simulink model "taller3"  (R2026a)
settings: Solver=VariableStepAuto  StopTime=20.0
libraries: simulink x2, slpidlib x1
settings Model: Creator=User  LastModifiedBy=User

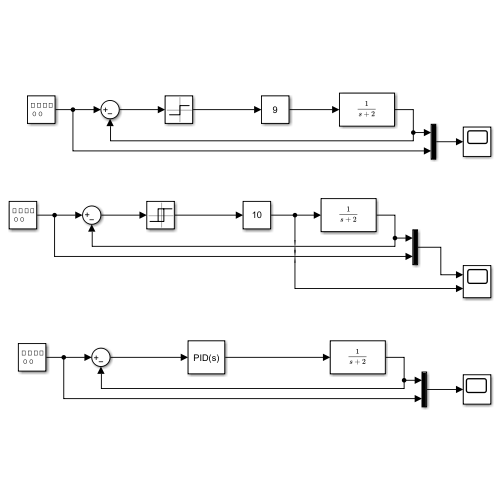
[thumbnail: Simulink's stored preview of the top-level diagram]
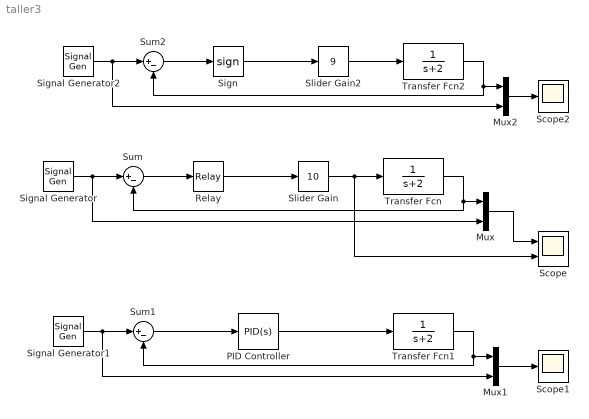
== system taller3 ==
  Mux : Mux  Inputs=2
  Mux1 : Mux  Inputs=2
  Mux2 : Mux  Inputs=2
  PID Controller : slpidlib/PID Controller  Controller=PID  Form=Parallel  TimeDomain=Continuous-time  UseExternalTs=off  SampleTime=-1  IntegratorMethod=Forward Euler  FilterMethod=Forward Euler  ControllerParametersSource=internal  P=50  I=0.5  UseKiTs=off  D=1  UseExternalDerivativeSource=off  N=100  UseFilter=on  TunerSelectOption=Transfer Function Based (PID Tuner App)  ZeroCross=off  InitialConditionSource=internal  InitialConditionForIntegrator=0  InitialConditionForFilter=0  DifferentiatorICPrevScaledInput=0  ExternalReset=none  TrackingMode=off  Kt=1  LimitOutput=off  SatLimitsSource=internal  UpperSaturationLimit=inf  LowerSaturationLimit=-inf  LinearizeAsGain=on  AntiWindupMode=none  Kb=1  LimitIntegrator=off  UpperIntegratorSaturationLimit=inf  LowerIntegratorSaturationLimit=-inf  POutMin=[]  POutMax=[]  IOutMin=[]  IOutMax=[]  DOutMin=[]  DOutMax=[]  NOutMin=[]  NOutMax=[]  SumOutMin=[]  SumOutMax=[]  SaturationOutMin=[]  SaturationOutMax=[]  PParamMin=[]  PParamMax=[]  IParamMin=[]  IParamMax=[]  DParamMin=[]  DParamMax=[]  NParamMin=[]  NParamMax=[]  KbParamMin=[]  KbParamMax=[]  KtParamMin=[]  KtParamMax=[]  KbOutMin=[]  KbOutMax=[]  KtOutMin=[]  KtOutMax=[]  IntegratorOutMin=[]  IntegratorOutMax=[]  FilterOutMin=[]  FilterOutMax=[]  SumI1OutMin=[]  SumI1OutMax=[]  SumI2OutMin=[]  SumI2OutMax=[]  SumI3OutMin=[]  SumI3OutMax=[]  SumI4OutMin=[]  SumI4OutMax=[]  SumDOutMin=[]  SumDOutMax=[]  DifferentiatorOutMin=[]  DifferentiatorOutMax=[]  FilterDiffOutCoefMin=[]  FilterDiffOutCoefMax=[]  ReciprocalOutMin=[]  ReciprocalOutMax=[]  SumDenOutMin=[]  SumDenOutMax=[]  SumNumOutMin=[]  SumNumOutMax=[]  DivideOutMin=[]  DivideOutMax=[]  UdiffTsProdOutMin=[]  UdiffTsProdOutMax=[]  NTsProdOutMin=[]  NTsProdOutMax=[]  UintegralTsProdOutMin=[]  UintegralTsProdOutMax=[]  UngainTsProdOutMin=[]  UngainTsProdOutMax=[]  ClampingZeroOutDataTypeStr=Inherit: Inherit via back propagation  ClampingZeroOutMin=[]  ClampingZeroOutMax=[]  FilterDenConstantOutDataTypeStr=Inherit: Inherit via back propagation  FilterDenConstantOutMin=[]  FilterDenConstantOutMax=[]  PCopyOutDataTypeStr=Inherit: Inherit via back propagation  PCopyOutMin=[]  PCopyOutMax=[]  NCopyOutDataTypeStr=Inherit: Inherit via back propagation  NCopyOutMin=[]  NCopyOutMax=[]  IntegratorContinuousStateAttributes=''  IntegratorStateMustResolveToSignalObject=off  IntegratorRTWStateStorageClass=Auto  FilterContinuousStateAttributes=''  FilterStateMustResolveToSignalObject=off  FilterRTWStateStorageClass=Auto  ParallelPVariant=InternalParameters  IdealPVariant=Disabled  IVariant=InternalParameters  DVariant=InternalParameters  IntegratorVariant=Continuous  SatVariant=Disabled  AWVariant=Passthrough  PCopyVariant=Disabled  TRVariant=Disabled  FdbkBlocksVariant=Forward  IdealPFdbkVariant=Disabled  SatFdbkVariant=Disabled  DerivativeFilterVariant=ContFilter  NVariant=InternalParameters  NCopyVariant=Disabled  FilterICVariant=InternalICsFilter  IntegratorICVariant=InternalICs  ExternalResetVariant=Disabled  TRSumVariant=Passthrough  SumFdbkVariant=Disabled  SumVariant=Sum_PID  TsampFilterVariant=InternalTs  TsampNgainVariant=Passthrough  TsampIntegralVariant=Disabled_SignalSpec  ExternalSaturationOutDataTypeStr=Inherit: Same as second input  DerivativeSourceVariant=ErrorSignal  PreIntVariant=InternalPreInt
  Relay : Relay  OnSwitchValue=0.2  OffSwitchValue=-0.2  OffOutputValue=-1
  Scope : Scope  NumInputPorts=2
      settings: ActiveDisplayYMinimum=-1.7321024139145964  ActiveDisplayYMaximum=2.2372388800155996
  Scope1 : Scope
      settings: ActiveDisplayYMinimum=-0.0268958546793987  ActiveDisplayYMaximum=1.0638458643477442
  Scope2 : Scope
      settings: ActiveDisplayYMinimum=-1.4990677225728488  ActiveDisplayYMaximum=1.847531136275848  DataLoggingVariableName=ScopeData2
  Sign : Signum  ZeroCross=off
  Signal Generator : SignalGenerator  WaveForm=square  Frequency=0.25
  Signal Generator1 : SignalGenerator  WaveForm=square  Frequency=0.25
  Signal Generator2 : SignalGenerator  WaveForm=square  Frequency=0.25
  Slider Gain : simulink/Math Operations/Slider Gain  gain=10  low=0  high=100
  Slider Gain2 : simulink/Math Operations/Slider Gain  gain=9  low=0  high=100
  Sum : Sum  Inputs=|+-
  Sum1 : Sum  Inputs=|+-
  Sum2 : Sum  Inputs=|+-
  Transfer Fcn : TransferFcn  Denominator=[1 2]
  Transfer Fcn1 : TransferFcn  Denominator=[1 2]
  Transfer Fcn2 : TransferFcn  Denominator=[1 2]
  wires:
  Signal Generator/1 -> Mux/2, Sum/1
  Transfer Fcn/1 -> Sum/2, Mux/1
  Mux/1 -> Scope/1
  Sum/1 -> Relay/1
  Relay/1 -> Slider Gain/1
  Slider Gain/1 -> Scope/2, Transfer Fcn/1
  PID Controller/1 -> Transfer Fcn1/1
  Transfer Fcn1/1 -> Sum1/2, Mux1/1
  Mux1/1 -> Scope1/1
  Sum1/1 -> PID Controller/1
  Signal Generator1/1 -> Mux1/2, Sum1/1
  Slider Gain2/1 -> Transfer Fcn2/1
  Transfer Fcn2/1 -> Sum2/2, Mux2/1
  Mux2/1 -> Scope2/1
  Sign/1 -> Slider Gain2/1
  Sum2/1 -> Sign/1
  Signal Generator2/1 -> Mux2/2, Sum2/1
